simulink model "Proyecto2017b"  (R2017b)
settings: Solver=VariableStepAuto  StartTime=0.0  StopTime=10.0  RelTol=1e-3
values from neighbouring files (symbols this model uses):
  b_h = b_eq_h * r_h ^ 2 / R_d ^ 2    (= 28800)    [automatas_matlab.m]
  b_t = b_eq_t * r_t ^ 2 / R_w_t ^ 2    (= 27000)    [automatas_matlab.m]
  b_w_h = 30000    [automatas_matlab.m]
  ba_h = M_h * n_h * w_pos_h    (= 864000)    [automatas_matlab.m]
  ba_t = M_t * n_t * w_pos_t    (= 810000)    [automatas_matlab.m]
  g = 9.80665    [automatas_matlab.m]
  k_bal = 10    [automatas_matlab.m]
  K_w_h = 1800000    [automatas_matlab.m]
  Ksa_h = M_h * n_h * w_pos_h^2    (= 5182464.45498)    [automatas_matlab.m]
  Ksa_t = M_t * n_t * w_pos_t^2    (= 3706277.11497)    [automatas_matlab.m]
  Ksia_h = M_h * w_pos_h ^ 3    (= 10361858.7296)    [automatas_matlab.m]
  Ksia_t = M_t * w_pos_t ^ 3    (= 5652876.56499)    [automatas_matlab.m]
  m_c = 50000    [automatas_matlab.m]
  M_h = (J_d + J_m_h * r_h ^ 2)/ R_d ^ 2    (= 48014.2222222)    [automatas_matlab.m]
  m_l = 65000    [automatas_matlab.m]
  M_t = m_c + (J_w_t + J_m_t * r_t ^ 2)/ R_w_t ^ 2    (= 59008)    [automatas_matlab.m]
  n_bal = 3    [automatas_matlab.m]
  R_d = 0.75    [automatas_matlab.m]
  r_h = 30    [automatas_matlab.m]
  r_t = 15    [automatas_matlab.m]
  R_w_t = 0.5    [automatas_matlab.m]
  x_t0 = 0    [automatas_matlab.m]
  y_t0 = 45    [automatas_matlab.m]    (also in crane.m; plot_crane.m; plot_crane_test.m)
libraries: simulink x2
settings Model: Creator=elust  LastModifiedBy=gonzalo
settings CodeAppCC: StateflowObjectComments=on

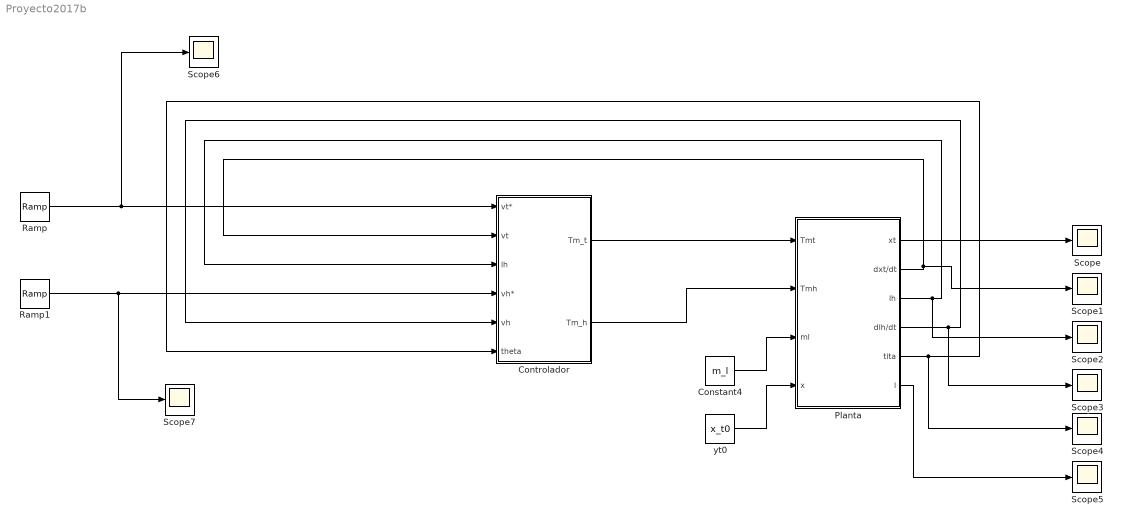
== system Proyecto2017b ==
  Constant4 : Constant  Value=m_l
  Controlador : Subsystem
  Planta : Subsystem
  Ramp : simulink/Sources/Ramp  slope=1  start=0  X0=0
  Ramp1 : simulink/Sources/Ramp  slope=1  start=0  X0=0
  Scope{,1..7} (8 alike) : Scope
  yt0 : Constant  Value=x_t0
  wires:
  Constant4/1 -> Planta/3(ml)
  Planta/1(xt) -> Scope/1
  Ramp/1 -> Scope6/1, Controlador/1(vt*)
  Planta/2(dxt/dt) -> Scope1/1, Controlador/2(vt)
  Planta/3(lh) -> Scope2/1, Controlador/3(lh)
  Planta/4(dlh/dt) -> Scope3/1, Controlador/5(vh)
  Planta/5(tita) -> Scope4/1, Controlador/6(theta)
  Controlador/1(Tm_t) -> Planta/1(Tmt)
  Controlador/2(Tm_h) -> Planta/2(Tmh)
  Planta/6(l) -> Scope5/1
  Ramp1/1 -> Scope7/1, Controlador/4(vh*)
  yt0/1 -> Planta/4(x)

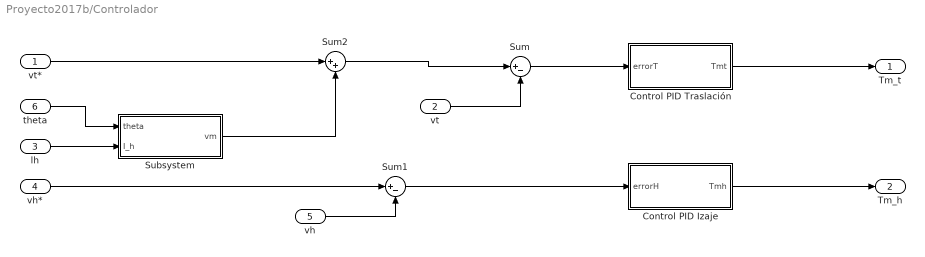
== system Proyecto2017b/Controlador ==
  vt* : Inport
  vt : Inport  Port=2
  lh : Inport  Port=3
  vh* : Inport  Port=4
  vh : Inport  Port=5
  theta : Inport  Port=6
  Control PID Izaje : Subsystem
  "Control PID Traslación " : Subsystem
  Subsystem : Subsystem
  Sum : Sum  Inputs=|+-
  Sum1 : Sum  Inputs=|+-
  Sum2 : Sum  Inputs=|++
  Tm_t : Outport
  Tm_h : Outport  Port=2
  wires:
  vt/1 -> Sum/2
  lh/1 -> Subsystem/2(I_h)
  theta/1 -> Subsystem/1(theta)
  Subsystem/1(vm) -> Sum2/2
  vt*/1 -> Sum2/1
  "Control PID Traslación "/1(Tmt) -> Tm_t/1
  vh*/1 -> Sum1/1
  Sum2/1 -> Sum/1
  Control PID Izaje/1(Tmh) -> Tm_h/1
  vh/1 -> Sum1/2
  Sum1/1 -> Control PID Izaje/1(errorH)
  Sum/1 -> "Control PID Traslación "/1(errorT)

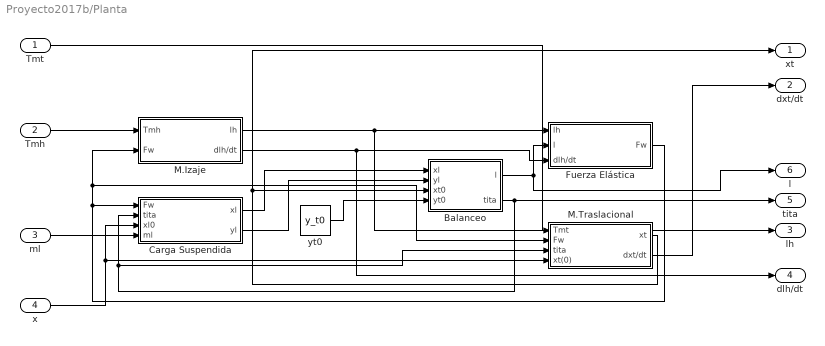
== system Proyecto2017b/Planta ==
  Tmt : Inport
  Tmh : Inport  Port=2
  ml : Inport  Port=3
  x : Inport  Port=4
  Balanceo : MATLAB Function  TreatAsAtomicUnit=on
  Carga Suspendida : Subsystem
  Fuerza Elástica : Subsystem
  M.Izaje : Subsystem
  M.Traslacional : Subsystem
  yt0 : Constant  Value=y_t0
  xt : Outport
  dxt/dt : Outport  Port=2
  lh : Outport  Port=3
  dlh/dt : Outport  Port=4
  tita : Outport  Port=5
  l : Outport  Port=6
  wires:
  ml/1 -> Carga Suspendida/4(ml)
  Carga Suspendida/1(xl) -> Balanceo/1(xl)
  M.Traslacional/2(dxt/dt) -> dxt/dt/1
  Fuerza Elástica/1(Fw) -> M.Izaje/2(Fw), M.Traslacional/2(Fw), Carga Suspendida/1(Fw)
  M.Traslacional/1(xt) -> xt/1, Balanceo/3(xt0)
  yt0/1 -> Balanceo/4(yt0)
  M.Izaje/2(dlh/dt) -> Fuerza Elástica/3(dlh/dt), dlh/dt/1
  M.Izaje/1(lh) -> Fuerza Elástica/1(lh), lh/1
  Tmh/1 -> M.Izaje/1(Tmh)
  Carga Suspendida/2(yl) -> Balanceo/2(yl)
  Balanceo/1(l) -> l/1, Fuerza Elástica/2(l)
  Balanceo/2(tita) -> tita/1, Carga Suspendida/2(tita), M.Traslacional/3(tita)
  Tmt/1 -> M.Traslacional/1("Tmt ")
  x/1 -> Carga Suspendida/3(xl0), M.Traslacional/4(xt(0))

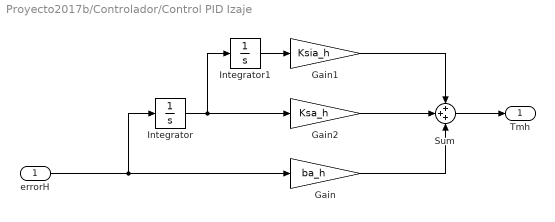
== system Proyecto2017b/Controlador/Control PID Izaje ==
  errorH : Inport
  Gain : Gain  Gain=ba_h
  Gain1 : Gain  Gain=Ksia_h
  Gain2 : Gain  Gain=Ksa_h
  Integrator : Integrator
  Integrator1 : Integrator
  Sum : Sum  Inputs=+++
  Tmh : Outport
  wires:
  Integrator1/1 -> Gain1/1
  errorH/1 -> Integrator/1, Gain/1
  Gain2/1 -> Sum/2
  Gain1/1 -> Sum/1
  Gain/1 -> Sum/3
  Sum/1 -> Tmh/1
  Integrator/1 -> Integrator1/1, Gain2/1

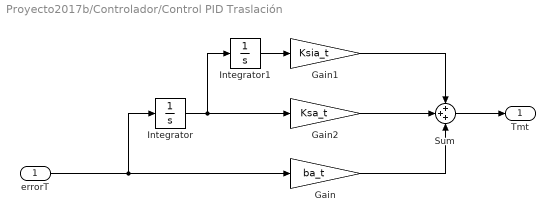
== system Proyecto2017b/Controlador/Control PID Traslación  ==
  errorT : Inport
  Gain : Gain  Gain=ba_t
  Gain1 : Gain  Gain=Ksia_t
  Gain2 : Gain  Gain=Ksa_t
  Integrator : Integrator
  Integrator1 : Integrator
  Sum : Sum  Inputs=+++
  Tmt : Outport
  wires:
  Integrator1/1 -> Gain1/1
  errorT/1 -> Integrator/1, Gain/1
  Gain2/1 -> Sum/2
  Gain1/1 -> Sum/1
  Gain/1 -> Sum/3
  Sum/1 -> Tmt/1
  Integrator/1 -> Integrator1/1, Gain2/1

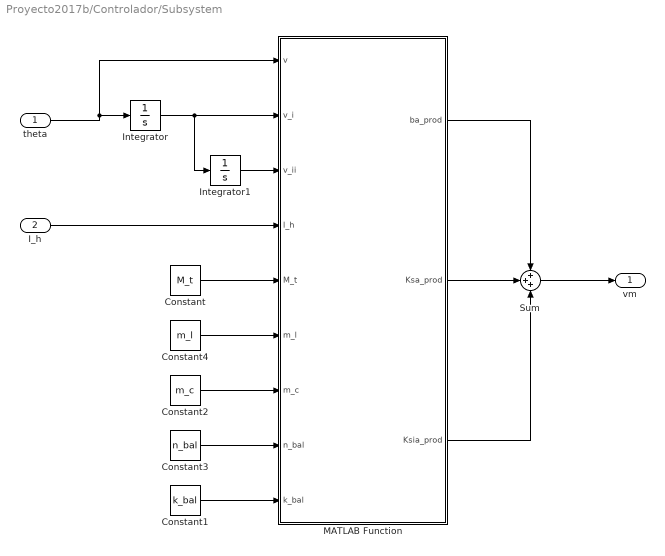
== system Proyecto2017b/Controlador/Subsystem ==
  theta : Inport
  I_h : Inport  Port=2
  Constant : Constant  Value=M_t
  Constant1 : Constant  Value=k_bal
  Constant2 : Constant  Value=m_c
  Constant3 : Constant  Value=n_bal
  Constant4 : Constant  Value=m_l
  Integrator : Integrator
  Integrator1 : Integrator
  MATLAB Function : MATLAB Function  TreatAsAtomicUnit=on
  Sum : Sum  Inputs=+++
  vm : Outport
  wires:
  MATLAB Function/1(ba_prod) -> Sum/1
  I_h/1 -> MATLAB Function/4(l_h)
  MATLAB Function/3(Ksia_prod) -> Sum/3
  MATLAB Function/2(Ksa_prod) -> Sum/2
  theta/1 -> Integrator/1, MATLAB Function/1(v)
  Integrator/1 -> Integrator1/1, MATLAB Function/2(v_i)
  Sum/1 -> vm/1
  Integrator1/1 -> MATLAB Function/3(v_ii)
  Constant/1 -> MATLAB Function/5(M_t)
  Constant2/1 -> MATLAB Function/7(m_c)
  Constant3/1 -> MATLAB Function/8(n_bal)
  Constant1/1 -> MATLAB Function/9(k_bal)
  Constant4/1 -> MATLAB Function/6(m_l)

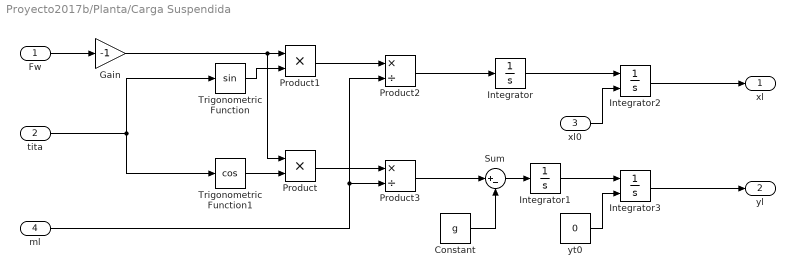
== system Proyecto2017b/Planta/Carga Suspendida ==
  Fw : Inport
  tita : Inport  Port=2
  xl0 : Inport  Port=3
  ml : Inport  Port=4
  Constant : Constant  Value=g
  Gain : Gain  Gain=-1
  Integrator : Integrator
  Integrator1 : Integrator
  Integrator2 : Integrator  InitialConditionSource=external
  Integrator3 : Integrator  InitialConditionSource=external
  Product : Product
  Product1 : Product
  Product2 : Product  Inputs=*/
  Product3 : Product  Inputs=*/
  Sum : Sum  Inputs=|+-
  Trigonometric Function : Trigonometry
  Trigonometric Function1 : Trigonometry  Operator=cos
  yt0 : Constant  Value=0
  xl : Outport
  yl : Outport  Port=2
  wires:
  tita/1 -> Trigonometric Function/1, Trigonometric Function1/1
  Constant/1 -> Sum/2
  Trigonometric Function1/1 -> Product/2
  Fw/1 -> Gain/1
  Trigonometric Function/1 -> Product1/2
  Sum/1 -> Integrator1/1
  Integrator/1 -> Integrator2/1
  Integrator1/1 -> Integrator3/1
  yt0/1 -> Integrator3/2
  xl0/1 -> Integrator2/2
  Integrator2/1 -> xl/1
  Integrator3/1 -> yl/1
  Product/1 -> Product3/1
  Product1/1 -> Product2/1
  ml/1 -> Product2/2, Product3/2
  Product2/1 -> Integrator/1
  Product3/1 -> Sum/1
  Gain/1 -> Product1/1, Product/1

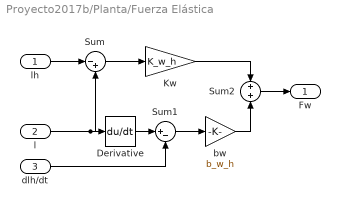
== system Proyecto2017b/Planta/Fuerza Elástica ==
  lh : Inport
  l : Inport  Port=2
  dlh/dt : Inport  Port=3
  Derivative : Derivative
  Kw : Gain  Gain=K_w_h
  Sum : Sum  Inputs=|-+
  Sum1 : Sum  Inputs=|+-
  Sum2 : Sum
  bw : Gain  Gain=b_w_h
  Fw : Outport
  wires:
  l/1 -> Sum/2, Derivative/1
  lh/1 -> Sum/1
  Sum/1 -> Kw/1
  Derivative/1 -> Sum1/1
  dlh/dt/1 -> Sum1/2
  Sum1/1 -> bw/1
  Sum2/1 -> Fw/1
  Kw/1 -> Sum2/1
  bw/1 -> Sum2/2

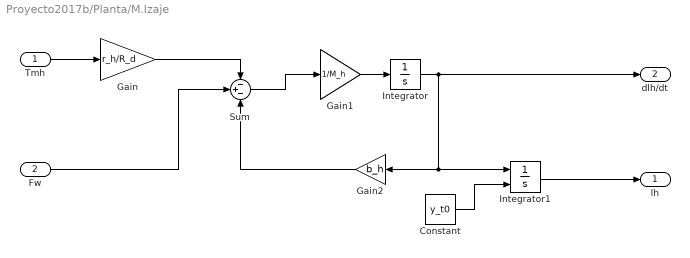
== system Proyecto2017b/Planta/M.Izaje ==
  Tmh : Inport
  Fw : Inport  Port=2
  Constant : Constant  Value=y_t0
  Gain : Gain  Gain=r_h/R_d
  Gain1 : Gain  Gain=1/M_h
  Gain2 : Gain  Gain=b_h
  Integrator : Integrator
  Integrator1 : Integrator  InitialConditionSource=external
  Sum : Sum  Inputs=-+-
  lh : Outport
  dlh/dt : Outport  Port=2
  wires:
  Tmh/1 -> Gain/1
  Gain/1 -> Sum/1
  Sum/1 -> Gain1/1
  Gain1/1 -> Integrator/1
  Integrator/1 -> dlh/dt/1, Integrator1/1, Gain2/1
  Gain2/1 -> Sum/3
  Fw/1 -> Sum/2
  Constant/1 -> Integrator1/2
  Integrator1/1 -> lh/1

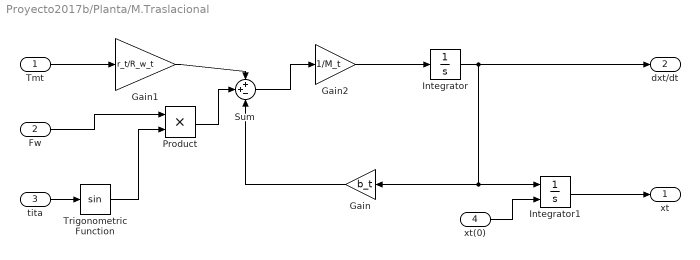
== system Proyecto2017b/Planta/M.Traslacional ==
  "Tmt " : Inport
  Fw : Inport  Port=2
  tita : Inport  Port=3
  xt(0) : Inport  Port=4
  Gain : Gain  Gain=b_t
  Gain1 : Gain  Gain=r_t/R_w_t
  Gain2 : Gain  Gain=1/M_t
  Integrator : Integrator
  Integrator1 : Integrator  InitialConditionSource=external
  Product : Product
  Sum : Sum  Inputs=++-
  Trigonometric Function : Trigonometry
  xt : Outport
  dxt/dt : Outport  Port=2
  wires:
  Gain2/1 -> Integrator/1
  Trigonometric Function/1 -> Product/2
  tita/1 -> Trigonometric Function/1
  Integrator/1 -> dxt/dt/1, Integrator1/1, Gain/1
  Gain/1 -> Sum/3
  Fw/1 -> Product/1
  Product/1 -> Sum/2
  Sum/1 -> Gain2/1
  Gain1/1 -> Sum/1
  xt(0)/1 -> Integrator1/2
  "Tmt "/1 -> Gain1/1
  Integrator1/1 -> xt/1

== matlab function Proyecto2017b/Controlador/Subsystem/MATLAB Function ==
  data: ba_prod output; Ksa_prod output; Ksia_prod output; v input; v_i input; v_ii input; l_h input; M_t input; m_l input; m_c input; n_bal input; k_bal input
function [ba_prod, Ksa_prod, Ksia_prod] = fcn(v, v_i, v_ii, l_h, M_t, m_l, m_c, n_bal, k_bal)


G_s = tf([-(m_c + m_l) 0],[(M_t + m_l) * l_h 0 M_t]);
poles = roots(G_s.den{1});

w_n = abs(poles(1));

w_pos = k_bal * w_n;

J_eq = - (M_t + m_l)/(m_c + m_l);

ba = J_eq * n_bal * w_pos;
Ksa = J_eq * n_bal * w_pos ^ 2;
Ksia = J_eq * w_pos ^ 3;


ba_prod = ba * v;
Ksa_prod = Ksa * v_i;
Ksia_prod = Ksia * v_ii;



end

== matlab function Proyecto2017b/Planta/Balanceo ==
  data: xl input; l output; yl input; xt0 input; yt0 input; tita output
function [l,tita] = fcn(xl,yl,xt0,yt0)

deltax = (xl - xt0);
deltay = (yl - yt0);


l = sqrt((deltax ^ 2) + (deltay ^ 2));

tita = atan2(deltax, deltay);

end
